simulink model "P702_NI_SoftECU"  (R2019a)
settings: Solver=ode1  StartTime=0.0  StopTime=Inf  FixedStep=0.001  RelTol=1e-3  EnableMultiTasking=on
PreLoadFcn:
  | run '.\VeriStand_BlockSet\NIVeriStandAddPaths.m'
undefined symbols (not defined in the file or in its folder): magnitude
libraries: simulink x83, simulink_extras x1
(part 41 of 76)

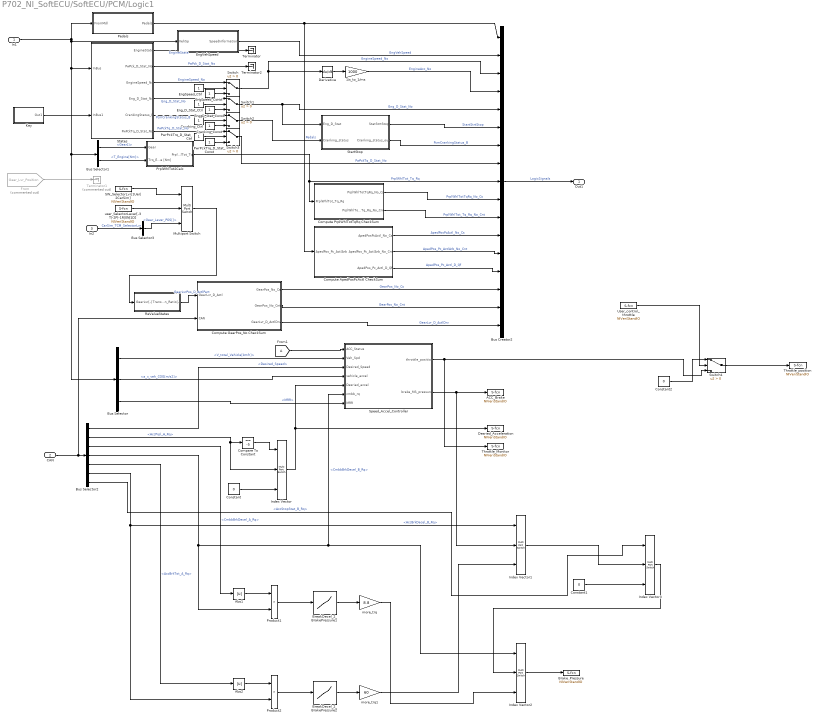
== system P702_NI_SoftECU/SoftECU/PCM/Logic1 ==
  In1 : Inport
  CAN : Inport  Port=2
  In2 : Inport  Port=3
  1/s_to_1/ms : Gain  Gain=1000
  ACC_Brake : S-Function  Priority=1  FunctionName=NIVeriStandIO  Parameters=width dtype portnum stime stype btype  SFunctionDeploymentMode=off  EnableBusSupport=off  mask(NI VeriStand Outport){portnum=1, width=-1, stime=-1, dtype=auto, stype=auto, btype=0}
      mask prompts: portnum "Port number:"; width "Port dimensions (-1 for dynamically sized):"; stime "Sample time (-1 for inherited):"; dtype "Data type:"; stype "Signal type:"; btype "Block type:"
      mask help: Use this outport on any level of nested subsystems to allow NI VeriStand software to map signals to it.
      mask init:
      | NIVeriStandIO_init;
      settings: CopyFcn=NIVeriStand_MDL_functions('', 'IO_copy');  DeleteFcn=NIVeriStand_MDL_functions('', 'IO_delete');  MoveFcn=set_param(gcb, 'Mask', 'on');
      mask Callback portnum: NIVeriStand_MDL_functions('', 'IO_setportnum');
      mask TypeOptions dtype: auto | double | single | int8 | uint8 | int16 | uint16 | int32 | uint32 | boolean
      mask Callback dtype: NIVeriStand_MDL_functions('', 'IO_booleansignal');
      mask TypeOptions stype: auto | real | complex
      mask Display:
      | patch([-x x], [-y y], [.90980 .81960 .32156]);
      | plot([xrad -x x xrad], [yrad -y y yrad]);
      | fprintf('NI Out%d', portnum);
  Abs1 : Abs
  Abs2 : Abs
  Brake_Pressure : S-Function  Priority=5  FunctionName=NIVeriStandIO  Parameters=width dtype portnum stime stype btype  SFunctionDeploymentMode=off  EnableBusSupport=off  mask(NI VeriStand Outport){portnum=5, width=-1, stime=-1, dtype=auto, stype=auto, btype=0}
      mask prompts: portnum "Port number:"; width "Port dimensions (-1 for dynamically sized):"; stime "Sample time (-1 for inherited):"; dtype "Data type:"; stype "Signal type:"; btype "Block type:"
      mask help: Use this outport on any level of nested subsystems to allow NI VeriStand software to map signals to it.
      mask init:
      | NIVeriStandIO_init;
      settings: CopyFcn=NIVeriStand_MDL_functions('', 'IO_copy');  DeleteFcn=NIVeriStand_MDL_functions('', 'IO_delete');  MoveFcn=set_param(gcb, 'Mask', 'on');
      mask Callback portnum: NIVeriStand_MDL_functions('', 'IO_setportnum');
      mask TypeOptions dtype: auto | double | single | int8 | uint8 | int16 | uint16 | int32 | uint32 | boolean
      mask Callback dtype: NIVeriStand_MDL_functions('', 'IO_booleansignal');
      mask TypeOptions stype: auto | real | complex
      mask Display:
      | patch([-x x], [-y y], [.90980 .81960 .32156]);
      | plot([xrad -x x xrad], [yrad -y y yrad]);
      | fprintf('NI Out%d', portnum);
  BreakDecel_2_BrakePressure1 : Lookup_n-D  NumberOfTableDimensions=1  BreakpointsForDimension1="[0   0.2  1   3.8   4.5    6     6.5   7   7.5   8   9   10    20]"  Table="[0   0.5    1   2       3     4      5      6   7     8    9   10   30]"  InternalRulePriority=Speed  RndMeth=Simplest  InputSameDT=on
  BreakDecel_2_BrakePressure2 : Lookup_n-D  NumberOfTableDimensions=1  BreakpointsForDimension1="[0   0.2  3.7   3.8   4.5    6     6.5   7   7.5   8   9   10    20]"  Table="[0   0    1   2       3     4      5      6   7     8    9   10   30]"  InternalRulePriority=Speed  RndMeth=Simplest  InputSameDT=on
  Bus Creator2 : BusCreator  Inputs=17
  Bus Selector : BusSelector  OutputSignals=V_total_Vehicle[km/h],a_x_veh_COG[m/s2],MRR
  Bus Selector1 : BusSelector  OutputSignals=Gear[],T_Engine[Nm]
  Bus Selector2 : BusSelector  OutputSignals=RealPCM.user_channel.Desired_Speed,ADAS.ACCDATA.AccPrpl_A_Rq,ADAS.ACCDATA_2.CmbbBrkDecel_A_Rq,ADAS.ACCDATA_2.CmbbBrkDecel_B_Rq,ADAS.ACCDATA.AccBrkTot_A_Rq,ADAS.ACCDATA.AccBrkDecel_B_Rq,ADAS.ACCDATA.AccStopStat_B_Rq
  Bus Selector3 : BusSelector  OutputSignals=Gear_Lever_POS[]
  Compare To Constant : simulink/Logic and Bit Operations/Compare To Constant  relop===  const=-5  OutDataTypeStr=boolean
  Compute ApedPosPcActl CheckSum : Subsystem
  Compute GearPos_No CheckSum : Subsystem
  Compute PrplWhlTotTqRq CheckSum : Subsystem
  Constant : Constant  Value=0
  Constant1 : Constant  Value=0
  Constant2 : Constant  Value=0
  Cranking_Const : Constant
  Cranking_Ctrl : Constant
  Derivative : Derivative
  Desried_Acceleration : S-Function  Priority=3  FunctionName=NIVeriStandIO  Parameters=width dtype portnum stime stype btype  SFunctionDeploymentMode=off  EnableBusSupport=off  mask(NI VeriStand Outport){portnum=3, width=-1, stime=-1, dtype=auto, stype=auto, btype=0}
      mask prompts: portnum "Port number:"; width "Port dimensions (-1 for dynamically sized):"; stime "Sample time (-1 for inherited):"; dtype "Data type:"; stype "Signal type:"; btype "Block type:"
      mask help: Use this outport on any level of nested subsystems to allow NI VeriStand software to map signals to it.
      mask init:
      | NIVeriStandIO_init;
      settings: CopyFcn=NIVeriStand_MDL_functions('', 'IO_copy');  DeleteFcn=NIVeriStand_MDL_functions('', 'IO_delete');  MoveFcn=set_param(gcb, 'Mask', 'on');
      mask Callback portnum: NIVeriStand_MDL_functions('', 'IO_setportnum');
      mask TypeOptions dtype: auto | double | single | int8 | uint8 | int16 | uint16 | int32 | uint32 | boolean
      mask Callback dtype: NIVeriStand_MDL_functions('', 'IO_booleansignal');
      mask TypeOptions stype: auto | real | complex
      mask Display:
      | patch([-x x], [-y y], [.90980 .81960 .32156]);
      | plot([xrad -x x xrad], [yrad -y y yrad]);
      | fprintf('NI Out%d', portnum);
  EngSpeed_Const : Constant
  EngSpeed_Ctrl : Constant
  EngVehSpeed : Subsystem
  Eng_D_Stat_Const : Constant
  Eng_D_Stat_Ctrl : Constant
  From : From  Commented=on  GotoTag=Gear_Lvr_Position  TagVisibility=global
  Index Vector{,1..3} (4 alike) : MultiPortSwitch  DataPortOrder=Zero-based contiguous  Inputs=2  zeroidx=on
  Key : Subsystem
      mask Display: disp('Key')
  Multiport Switch : MultiPortSwitch  Inputs=2
  Pedals : Subsystem
  Product1 : Product
  Product2 : Product
  PrplWhlTot2Calc : Subsystem
  PwrPckTrq_D_Stat_Const : Constant
  PwrPckTrq_D_Stat_Ctrl : Constant
  ReValueStates : Subsystem
      mask Display: disp('RevalueStates')
  SW_SelectorLvr[1Uer|2CarSim] : S-Function  Priority=2  FunctionName=NIVeriStandIO  Parameters=width dtype portnum stime stype btype  SFunctionDeploymentMode=off  EnableBusSupport=off  mask(NI VeriStand Inport){portnum=2, width=-1, stime=-1, dtype=auto, stype=auto, btype=1}
      mask prompts: portnum "Port number:"; width "Port dimensions (-1 for dynamically sized):"; stime "Sample time (-1 for inherited):"; dtype "Data type:"; stype "Signal type:"; btype "Block type:"
      mask help: Use this inport on any level of nested subsystems to allow NI VeriStand software to map signals to it.
      mask init:
      | NIVeriStandIO_init;
      settings: CopyFcn=NIVeriStand_MDL_functions('', 'IO_copy');  DeleteFcn=NIVeriStand_MDL_functions('', 'IO_delete');  MoveFcn=set_param(gcb, 'Mask', 'on');
      mask Callback portnum: NIVeriStand_MDL_functions('', 'IO_setportnum');
      mask TypeOptions dtype: auto | double | single | int8 | uint8 | int16 | uint16 | int32 | uint32 | boolean
      mask Callback dtype: NIVeriStand_MDL_functions('', 'IO_booleansignal');
      mask TypeOptions stype: auto | real | complex
      mask Display:
      | patch([-x x], [-y y], [.90980 .81960 .32156]);
      | plot([xrad -x x xrad], [yrad -y y yrad]);
      | fprintf('NI In%d', portnum);
  Speed_Accel_Controller : Subsystem
  StartStop : Subsystem
  States : Subsystem
  Switch{,1..4} (5 alike) : Switch  Criteria=u2 > Threshold
  Terminator : Terminator
  Terminator1 : Terminator  Commented=on
  Terminator2 : Terminator
  Throttle_Monitor : S-Function  Priority=4  FunctionName=NIVeriStandIO  Parameters=width dtype portnum stime stype btype  SFunctionDeploymentMode=off  EnableBusSupport=off  mask(NI VeriStand Outport){portnum=4, width=-1, stime=-1, dtype=auto, stype=auto, btype=0}
      mask prompts: portnum "Port number:"; width "Port dimensions (-1 for dynamically sized):"; stime "Sample time (-1 for inherited):"; dtype "Data type:"; stype "Signal type:"; btype "Block type:"
      mask help: Use this outport on any level of nested subsystems to allow NI VeriStand software to map signals to it.
      mask init:
      | NIVeriStandIO_init;
      settings: CopyFcn=NIVeriStand_MDL_functions('', 'IO_copy');  DeleteFcn=NIVeriStand_MDL_functions('', 'IO_delete');  MoveFcn=set_param(gcb, 'Mask', 'on');
      mask Callback portnum: NIVeriStand_MDL_functions('', 'IO_setportnum');
      mask TypeOptions dtype: auto | double | single | int8 | uint8 | int16 | uint16 | int32 | uint32 | boolean
      mask Callback dtype: NIVeriStand_MDL_functions('', 'IO_booleansignal');
      mask TypeOptions stype: auto | real | complex
      mask Display:
      | patch([-x x], [-y y], [.90980 .81960 .32156]);
      | plot([xrad -x x xrad], [yrad -y y yrad]);
      | fprintf('NI Out%d', portnum);
  Throttle_position : S-Function  Priority=2  FunctionName=NIVeriStandIO  Parameters=width dtype portnum stime stype btype  SFunctionDeploymentMode=off  EnableBusSupport=off  mask(NI VeriStand Outport){portnum=2, width=-1, stime=-1, dtype=auto, stype=auto, btype=0}
      mask prompts: portnum "Port number:"; width "Port dimensions (-1 for dynamically sized):"; stime "Sample time (-1 for inherited):"; dtype "Data type:"; stype "Signal type:"; btype "Block type:"
      mask help: Use this outport on any level of nested subsystems to allow NI VeriStand software to map signals to it.
      mask init:
      | NIVeriStandIO_init;
      settings: CopyFcn=NIVeriStand_MDL_functions('', 'IO_copy');  DeleteFcn=NIVeriStand_MDL_functions('', 'IO_delete');  MoveFcn=set_param(gcb, 'Mask', 'on');
      mask Callback portnum: NIVeriStand_MDL_functions('', 'IO_setportnum');
      mask TypeOptions dtype: auto | double | single | int8 | uint8 | int16 | uint16 | int32 | uint32 | boolean
      mask Callback dtype: NIVeriStand_MDL_functions('', 'IO_booleansignal');
      mask TypeOptions stype: auto | real | complex
      mask Display:
      | patch([-x x], [-y y], [.90980 .81960 .32156]);
      | plot([xrad -x x xrad], [yrad -y y yrad]);
      | fprintf('NI Out%d', portnum);
  User_control_throttle : S-Function  Priority=3  FunctionName=NIVeriStandIO  Parameters=width dtype portnum stime stype btype  SFunctionDeploymentMode=off  EnableBusSupport=off  mask(NI VeriStand Inport){portnum=3, width=-1, stime=-1, dtype=auto, stype=auto, btype=1}
      mask prompts: portnum "Port number:"; width "Port dimensions (-1 for dynamically sized):"; stime "Sample time (-1 for inherited):"; dtype "Data type:"; stype "Signal type:"; btype "Block type:"
      mask help: Use this inport on any level of nested subsystems to allow NI VeriStand software to map signals to it.
      mask init:
      | NIVeriStandIO_init;
      settings: CopyFcn=NIVeriStand_MDL_functions('', 'IO_copy');  DeleteFcn=NIVeriStand_MDL_functions('', 'IO_delete');  MoveFcn=set_param(gcb, 'Mask', 'on');
      mask Callback portnum: NIVeriStand_MDL_functions('', 'IO_setportnum');
      mask TypeOptions dtype: auto | double | single | int8 | uint8 | int16 | uint16 | int32 | uint32 | boolean
      mask Callback dtype: NIVeriStand_MDL_functions('', 'IO_booleansignal');
      mask TypeOptions stype: auto | real | complex
      mask Display:
      | patch([-x x], [-y y], [.90980 .81960 .32156]);
      | plot([xrad -x x xrad], [yrad -y y yrad]);
      | fprintf('NI In%d', portnum);
  more_trq : Gain  Gain=8.8
  more_trq1 : Gain  Gain=60
  user_SelectorLever[-3T|-2P|-1R|0N|1D] : S-Function  Priority=1  FunctionName=NIVeriStandIO  Parameters=width dtype portnum stime stype btype  SFunctionDeploymentMode=off  EnableBusSupport=off  mask(NI VeriStand Inport){portnum=1, width=-1, stime=-1, dtype=auto, stype=auto, btype=1}
      mask prompts: portnum "Port number:"; width "Port dimensions (-1 for dynamically sized):"; stime "Sample time (-1 for inherited):"; dtype "Data type:"; stype "Signal type:"; btype "Block type:"
      mask help: Use this inport on any level of nested subsystems to allow NI VeriStand software to map signals to it.
      mask init:
      | NIVeriStandIO_init;
      settings: CopyFcn=NIVeriStand_MDL_functions('', 'IO_copy');  DeleteFcn=NIVeriStand_MDL_functions('', 'IO_delete');  MoveFcn=set_param(gcb, 'Mask', 'on');
      mask Callback portnum: NIVeriStand_MDL_functions('', 'IO_setportnum');
      mask TypeOptions dtype: auto | double | single | int8 | uint8 | int16 | uint16 | int32 | uint32 | boolean
      mask Callback dtype: NIVeriStand_MDL_functions('', 'IO_booleansignal');
      mask TypeOptions stype: auto | real | complex
      mask Display:
      | patch([-x x], [-y y], [.90980 .81960 .32156]);
      | plot([xrad -x x xrad], [yrad -y y yrad]);
      | fprintf('NI In%d', portnum);
  Out1 : Outport
  wires:
  Key/1(Out1) -> States/2(InBus1)
  ReValueStates/1(Transmission_Ratio[-]) -> Compute GearPos_No CheckSum/1(GearLvr_D_Actl)  "GearLvrPos_D_ActlPart"
  From/1 -> Terminator1/1
  Switch3/1 -> Bus Creator2/8  "PwPckTq_D_Stat_No"
  States/6(PwPckTq_D_Stat_No) -> Switch3/1  "PwPckTq_D_Stat_No"
  PwrPckTrq_D_Stat_Ctrl/1 -> Switch3/2
  PwrPckTrq_D_Stat_Const/1 -> Switch3/3
  Switch2/1 -> StartStop/2(Cranking_status)
  Cranking_Ctrl/1 -> Switch2/2
  Cranking_Const/1 -> Switch2/3
  Eng_D_Stat_Ctrl/1 -> Switch1/2
  Eng_D_Stat_Const/1 -> Switch1/3
  Switch1/1 -> StartStop/1(Eng_D_Stat), Bus Creator2/5  "Eng_D_Stat_No"
  EngSpeed_Ctrl/1 -> Switch/2
  EngSpeed_Const/1 -> Switch/3
  Switch/1 -> Bus Creator2/3, Derivative/1  "EngineSpeed_No"
  States/5(CrankingStatus_B) -> Switch2/1  "PcmCrankingStatus_B"
  States/4(Eng_D_Stat_No) -> Switch1/1  "Eng_D_Stat_No"
  States/3(EngineSpeed_No) -> Switch/1  "EngineSpeed_No"
  PrplWhlTot2Calc/1(PrplWhlTot_Tq) -> Compute PrplWhlTotTqRq CheckSum/1(PrplWhlTot_Tq_Rq), Bus Creator2/9  "PrplWhlTot_Tq_Rq"
  Bus Selector1/2 -> PrplWhlTot2Calc/2(Trq_Engine [Nm])  "<T_Engine[Nm]>"
  Bus Selector1/1 -> PrplWhlTot2Calc/1(Gear)  "<Gear[]>"
  In1/1 -> Bus Selector/1, Bus Selector1/1, States/1(InBus), EngVehSpeed/1(VehSp), Pedals/1(FromMdl)
  EngVehSpeed/1(SpeedInformation) -> Bus Creator2/2  "EngVehSpeed"
  Pedals/1(Pedals) -> Compute ApedPosPcActl CheckSum/1(ApedPos_Pc_ActlArb), Bus Creator2/1  "Pedals"
  StartStop/2(Cranking_status_out) -> Bus Creator2/7  "PcmCrankingStatus_B"
  StartStop/1(StatStrtStop) -> Bus Creator2/6  "StartStrtStop"
  1/s_to_1/ms/1 -> Bus Creator2/4  "EngineAcc_No"
  Derivative/1 -> 1/s_to_1/ms/1
  Bus Creator2/1 -> Out1/1  "LogicSignals"
  States/2("PwPck_D_Stat_No ") -> Terminator2/1  "PwPck_D_Stat_No"
  States/1(EngineState) -> Terminator/1  "EngineState"
  Compute PrplWhlTotTqRq CheckSum/1(PrplWhlTotTqRq_No_Cs) -> Bus Creator2/10  "PrplWhlTotTqRq_No_Cs"
  Compute ApedPosPcActl CheckSum/1(ApedPosPcActl_No_Cs) -> Bus Creator2/12  "ApedPosPcActl_No_Cs"
  Compute PrplWhlTotTqRq CheckSum/2(PrplWhlTot_Tq_Rq_No_Cnt) -> Bus Creator2/11  "PrplWhlTot_Tq_Rq_No_Cnt"
  Compute ApedPosPcActl CheckSum/3(ApedPos_Pc_Actl_D_Qf) -> Bus Creator2/14  "ApedPos_Pc_Actl_D_Qf"
  Compute ApedPosPcActl CheckSum/2(ApedPos_Pc_ActlArb_No_Cnt) -> Bus Creator2/13  "ApedPos_Pc_ActlArb_No_Cnt"
  Compute GearPos_No CheckSum/3(GearLvr_D_ActlDrv) -> Bus Creator2/17  "GearLvr_D_ActlDrv"
  Compute GearPos_No CheckSum/2(GearPos_No_Cnt) -> Bus Creator2/16  "GearPos_No_Cnt"
  Compute GearPos_No CheckSum/1(GearPos_No_Cs) -> Bus Creator2/15  "GearPos_No_Cs"
  CAN/1 -> Compute GearPos_No CheckSum/2(CAN), Bus Selector2/1
  Speed_Accel_Controller/1(throttle_position) -> Switch4/3, Throttle_Monitor/1
  Bus Selector/1 -> Speed_Accel_Controller/2(Veh_Spd)  "<V_total_Vehicle[km/h]>"
  Bus Selector2/1 -> Speed_Accel_Controller/3(Desired_Speed)  "<Desired_Speed>"
  Bus Selector/2 -> Speed_Accel_Controller/4(vehicle_accel)  "<a_x_veh_COG[m/s2]>"
  [A] -> Speed_Accel_Controller/1(ACC_Status)
  Bus Selector2/5 -> Abs2/1  "<AccBrkTot_A_Rq>"
  Bus Selector2/2 -> Index Vector/2, Compare To Constant/1  "<AccPrpl_A_Rq>"
  Compare To Constant/1 -> Index Vector/1
  Constant/1 -> Index Vector/3
  Index Vector/1 -> Speed_Accel_Controller/5(Desried_accel), Desried_Acceleration/1
  Speed_Accel_Controller/2(brake_MS_pressure) -> Index Vector1/2, ACC_Brake/1
  Bus Selector2/4 -> Speed_Accel_Controller/6(cmbb_rq), Index Vector2/1, Product1/2  "<CmbbBrkDecel_B_Rq>"
  BreakDecel_2_BrakePressure1/1 -> more_trq/1
  Product1/1 -> BreakDecel_2_BrakePressure1/1
  Abs1/1 -> Product1/1
  Bus Selector2/3 -> Abs1/1  "<CmbbBrkDecel_A_Rq>"
  BreakDecel_2_BrakePressure2/1 -> more_trq1/1
  Product2/1 -> BreakDecel_2_BrakePressure2/1
  Abs2/1 -> Product2/1
  more_trq1/1 -> Index Vector1/3
  Bus Selector2/6 -> Index Vector1/1, Product2/2  "<AccBrkDecel_B_Rq>"
  Index Vector3/1 -> Index Vector2/2
  more_trq/1 -> Index Vector2/3
  Index Vector2/1 -> Brake_Pressure/1
  Index Vector1/1 -> Index Vector3/2
  Bus Selector2/7 -> Index Vector3/1  "<AccStopStat_B_Rq>"
  Constant1/1 -> Index Vector3/3
  Constant2/1 -> Switch4/1
  Switch4/1 -> Throttle_position/1
  Bus Selector/3 -> Speed_Accel_Controller/7(MRR)  "<MRR>"
  user_SelectorLever[-3T|-2P|-1R|0N|1D]/1 -> Multiport Switch/2
  Multiport Switch/1 -> ReValueStates/1(GearLvr[-])
  SW_SelectorLvr[1Uer|2CarSim]/1 -> Multiport Switch/1
  In2/1 -> Bus Selector3/1  "CarSim_TCM_SelectorLvr"
  Bus Selector3/1 -> Multiport Switch/3  "<Gear_Lever_POS[]>"
  User_control_throttle/1 -> Switch4/2

== system P702_NI_SoftECU/SoftECU/PCM/Mapping ==
  In1 : Inport
  Bus Creator : BusCreator  Inputs=9
  EngBrakeData : Subsystem
  EngVehicleSpThrottle : Subsystem
  EngVehicleSpThrottle2 : Subsystem
  EngineClimateData : Subsystem
  EngineClutchData : Subsystem
  EngineData_7 : Subsystem
  PowertrainData_10 : Subsystem
  TorqueDataEngFlags : Subsystem
  VehicleOperatingModes : Subsystem
  Out1 : Outport
  wires:
  TorqueDataEngFlags/1(Out1) -> Bus Creator/8  "TorqueDataEngFlags"
  EngineData_7/1(Out1) -> Bus Creator/7  "EngineData_7"
  VehicleOperatingModes/1(Out1) -> Bus Creator/6  "VehicleOperatingModes"
  EngVehicleSpThrottle2/1(Out1) -> Bus Creator/5  "EngVehicleSpThottle2"
  EngVehicleSpThrottle/1(Out1) -> Bus Creator/4  "EngVehicleSpThrottle"
  EngineClutchData/1(Out1) -> Bus Creator/3  "EngineClutchData"
  EngineClimateData/1(Out1) -> Bus Creator/2  "EngineClimateData"
  EngBrakeData/1(Out1) -> Bus Creator/1  "EngBrakeData"
  Bus Creator/1 -> Out1/1  "MsgSignals"
  In1/1 -> EngBrakeData/1(In1), EngineClimateData/1(In1), EngineClutchData/1(In1), EngVehicleSpThrottle/1(In1), EngineData_7/1(In1), PowertrainData_10/1(In1), TorqueDataEngFlags/1(In1), VehicleOperatingModes/1(In1), EngVehicleSpThrottle2/1(In1)
  PowertrainData_10/1(Out1) -> Bus Creator/9  "PowertrainData_10"

== system P702_NI_SoftECU/SoftECU/PSCM/Logic ==
  In1 : Inport
  Bus Creator : BusCreator  Inputs=3
  Checksums : Subsystem
  Counters : Subsystem
  UnitConversion : Subsystem
  Out1 : Outport
  wires:
  In1/1 -> UnitConversion/1(In1)
  Bus Creator/1 -> Out1/1  "LogicSignals"
  UnitConversion/1(Out1) -> Bus Creator/1, Checksums/4(StePinRelCalib_Sns), Checksums/3(StePinComp_Est), Checksums/2(StePinRelInit_Sns)
  Counters/1(Out1) -> Checksums/1(StePinAng_Counter), Bus Creator/2
  Checksums/1(Out1) -> Bus Creator/3

== system P702_NI_SoftECU/SoftECU/PSCM/Mapping ==
  In1 : Inport
  SteeringPinion_Data : Subsystem
  Out1 : Outport
  wires:
  SteeringPinion_Data/1(Out1) -> Out1/1
  In1/1 -> SteeringPinion_Data/1(In1)

== system P702_NI_SoftECU/SoftECU/RCM/Logic ==
  In1 : Inport
  Bus Creator : BusCreator  Inputs=4
  Bus Selector : BusSelector  OutputSignals=RollRate_Vehicle_CoG[rad|s],YawRate_Vehicle_CoG[rad|s],a_y_Vehicle_CoG[m|s2],a_x_Vehicle_CoG[m|s2],a_z_Vehicle_CoG[m|s2]
  Bus Selector1 : BusSelector  OutputSignals=RollYawCounter,AccelCounter
  Checksums : Subsystem
  Counters : Subsystem
  StatusMessage : Subsystem
  UnitConversion : Subsystem
  Out1 : Outport
  wires:
  In1/1 -> UnitConversion/1(In1), StatusMessage/1(In1)
  Bus Creator/1 -> Out1/1  "LogicSignals"
  UnitConversion/1(Out1) -> Bus Selector/1, Bus Creator/1
  StatusMessage/1(Out1) -> Bus Creator/2
  Counters/1(Out1) -> Bus Creator/3, Bus Selector1/1
  Checksums/1(Out1) -> Bus Creator/4
  Bus Selector/1 -> Checksums/3(RollRate)  "<RollRate_Vehicle_CoG[rad|s]>"
  Bus Selector/2 -> Checksums/4(YawRate)  "<YawRate_Vehicle_CoG[rad|s]>"
  Bus Selector1/1 -> Checksums/1(Counter)  "<RollYawCounter>"
  Bus Selector1/2 -> Checksums/2(Accel_Counter)  "<AccelCounter>"
  Bus Selector/4 -> Checksums/6(LongAccel)  "<a_x_Vehicle_CoG[m|s2]>"
  Bus Selector/3 -> Checksums/5(LatAccel)  "<a_y_Vehicle_CoG[m|s2]>"
  Bus Selector/5 -> Checksums/7(VertAccel)  "<a_z_Vehicle_CoG[m|s2]>"

== system P702_NI_SoftECU/SoftECU/RCM/Mapping ==
  In1 : Inport
  Accel_Data : Subsystem
  Bus Creator : BusCreator  Inputs=3
  RCMStatusMessage2 : Subsystem
  Yaw_Data : Subsystem
  Out1 : Outport
  wires:
  Bus Creator/1 -> Out1/1  "MsgSignals"
  In1/1 -> Accel_Data/1(In1), Yaw_Data/1(In1), RCMStatusMessage2/1(In1)
  Accel_Data/1(Out1) -> Bus Creator/1  "Accel_Data"
  Yaw_Data/1(Out1) -> Bus Creator/2  "Yaw_Data"
  RCMStatusMessage2/1(Out1) -> Bus Creator/3

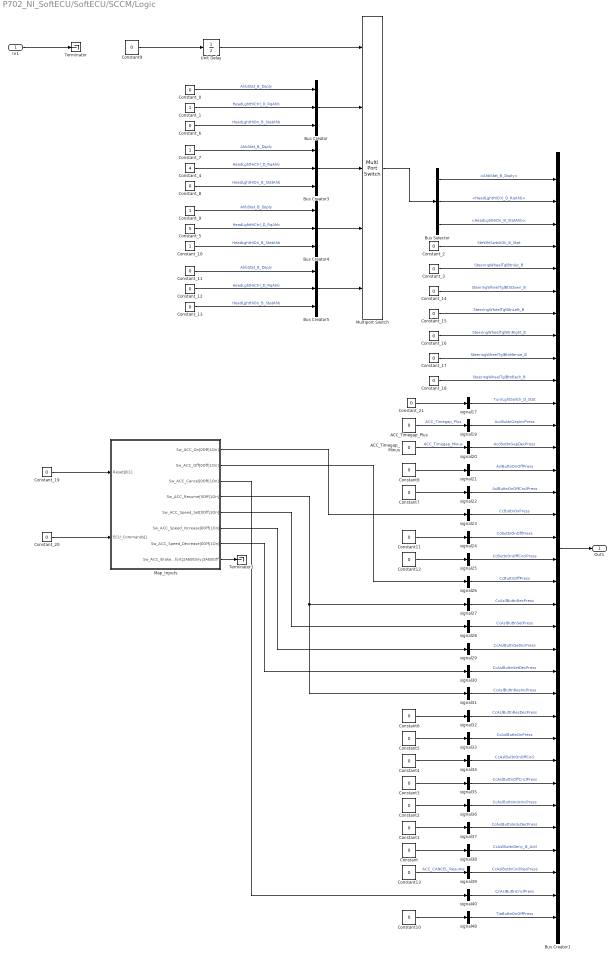
== system P702_NI_SoftECU/SoftECU/SCCM/Logic ==
  In1 : Inport
  ACC_Timegap_Minus : Constant  Value=0
  ACC_Timegap_Plus : Constant  Value=0
  Bus Creator{,3..5} (4 alike) : BusCreator  Inputs=3
  Bus Creator1 : BusCreator  Inputs=34
  Bus Selector : BusSelector  OutputSignals=AhbStat_B_Dsply,HeadLghtHiCtrl_D_RqAhb,HeadLghtHiOn_B_StatAhb
  Constant{,1..9,11..13} (13 alike) : Constant  Value=0
  Constant10 : Constant  Value=0  OutDataTypeStr=boolean
  Constant_{0,2..3,6,8,11..21} (16 alike) : Constant  Value=0
  Constant_{1,7,9..10} (4 alike) : Constant
  Constant_4 : Constant  Value=4
  Constant_5 : Constant  Value=5
  Map_Inputs : Subsystem
  Multiport Switch : MultiPortSwitch  DataPortOrder=Zero-based contiguous  Inputs=4  zeroidx=on
  Terminator : Terminator
  Terminator1 : Terminator
  Unit Delay : UnitDelay  SampleTime=-1  HasFrameUpgradeWarning=on
  signal{17,19..40,48} (24 alike) : Demux  Outputs=1
  Out1 : Outport
  wires:
  Constant9/1 -> Unit Delay/1
  Constant_0/1 -> Bus Creator/1  "AhbStat_B_Dsply"
  Constant_1/1 -> Bus Creator/2  "HeadLghtHiCtrl_D_RqAhb"
  Constant_6/1 -> Bus Creator/3  "HeadLghtHiOn_B_StatAhb"
  Bus Creator/1 -> Multiport Switch/2
  Constant_7/1 -> Bus Creator3/1  "AhbStat_B_Dsply"
  Constant_4/1 -> Bus Creator3/2  "HeadLghtHiCtrl_D_RqAhb"
  Constant_8/1 -> Bus Creator3/3  "HeadLghtHiOn_B_StatAhb"
  Bus Creator3/1 -> Multiport Switch/3
  Constant_9/1 -> Bus Creator4/1  "AhbStat_B_Dsply"
  Constant_5/1 -> Bus Creator4/2  "HeadLghtHiCtrl_D_RqAhb"
  Constant_10/1 -> Bus Creator4/3  "HeadLghtHiOn_B_StatAhb"
  Bus Creator4/1 -> Multiport Switch/4
  Constant_11/1 -> Bus Creator5/1  "AhbStat_B_Dsply"
  Constant_12/1 -> Bus Creator5/2  "HeadLghtHiCtrl_D_RqAhb"
  Constant_13/1 -> Bus Creator5/3  "HeadLghtHiOn_B_StatAhb"
  Bus Creator5/1 -> Multiport Switch/5
  Unit Delay/1 -> Multiport Switch/1
  Multiport Switch/1 -> Bus Selector/1
  Bus Selector/1 -> Bus Creator1/1  "<AhbStat_B_Dsply>"
  Bus Selector/2 -> Bus Creator1/2  "<HeadLghtHiCtrl_D_RqAhb>"
  Bus Selector/3 -> Bus Creator1/3  "<HeadLghtHiOn_B_StatAhb>"
  Bus Creator1/1 -> Out1/1
  Constant_2/1 -> Bus Creator1/4  "SteWhlSwtchOk_B_Stat"
  Constant_3/1 -> Bus Creator1/5  "SteeringWheelTglBtnUp_B"
  Constant_15/1 -> Bus Creator1/7  "SteeringWheelTglBtnLeft_B"
  Constant_16/1 -> Bus Creator1/8  "SteeringWheelTglBtnRight_B"
  Constant_17/1 -> Bus Creator1/9  "SteeringWheelTglBtnMenue_B"
  Constant_18/1 -> Bus Creator1/10  "SteeringWheelTglBtnBack_B"
  Constant_14/1 -> Bus Creator1/6  "SteeringWheelTglBtnDown_B"
  Constant10/1 -> signal48/1
  signal48/1 -> Bus Creator1/34  "TjaButtnOnOffPress"
  In1/1 -> Terminator/1
  signal40/1 -> Bus Creator1/33  "CcAslButtnCnclPress"
  signal39/1 -> Bus Creator1/32  "CcAslButtnCnclResPress"
  Constant/1 -> signal38/1
  signal38/1 -> Bus Creator1/31  "CcAslButtnDeny_B_Actl"
  Constant1/1 -> signal37/1
  signal37/1 -> Bus Creator1/30  "CcAslButtnIndxDecPress"
  Constant2/1 -> signal36/1
  signal36/1 -> Bus Creator1/29  "CcAslButtnIndxIncPress"
  Constant3/1 -> signal35/1
  signal35/1 -> Bus Creator1/28  "CcAslButtnOffCnclPress"
  Constant4/1 -> signal34/1
  signal34/1 -> Bus Creator1/27  "CcAslButtnOnOffCncl"
  Constant5/1 -> signal33/1
  signal33/1 -> Bus Creator1/26  "CcAslButtnOnPress"
  Constant6/1 -> signal32/1
  signal32/1 -> Bus Creator1/25  "CcAslButtnResDecPress"
  signal31/1 -> Bus Creator1/24  "CcAslButtnResIncPress"
  signal30/1 -> Bus Creator1/23  "CcAslButtnSetDecPress"
  signal29/1 -> Bus Creator1/22  "CcAslButtnSetIncPress"
  Map_Inputs/5(Sw_ACC_Speed_Set[0Off|1On]) -> signal28/1
  signal28/1 -> Bus Creator1/21  "CcAslButtnSetPress"
  signal27/1 -> Bus Creator1/20  "CcAsllButtnResPress"
  signal26/1 -> Bus Creator1/19  "CcButtnOffPress"
  signal25/1 -> Bus Creator1/18  "CcButtnOnOffCnclPress"
  Constant7/1 -> signal22/1
  Constant8/1 -> signal21/1
  Constant_21/1 -> signal17/1
  ACC_Timegap_Plus/1 -> signal19/1  "ACC_Timegap_Plus"
  Map_Inputs/1(Sw_ACC_On[0Off|1On]) -> signal23/1
  Constant11/1 -> signal24/1
  Map_Inputs/2(Sw_ACC_Off[0Off|1On]) -> signal26/1
  Map_Inputs/4(Sw_ACC_Resume[0Off|1On]) -> signal27/1, signal31/1
  Map_Inputs/6(Sw_ACC_Speed_Increase[0Off|1On]) -> signal29/1
  Map_Inputs/7(Sw_ACC_Speed_Decrease[0Off|1On]) -> signal30/1
  Constant13/1 -> signal39/1  "ACC_CANCEL_Resume"
  Map_Inputs/3(Sw_ACC_Cancel[0Off|1On]) -> signal40/1
  signal24/1 -> Bus Creator1/17  "CcButtnOnOffPress"
  signal23/1 -> Bus Creator1/16  "CcButtnOnPress"
  signal22/1 -> Bus Creator1/15  "AslButtnOnOffCnclPress"
  signal21/1 -> Bus Creator1/14  "AslButtnOnOffPress"
  signal20/1 -> Bus Creator1/13  "AccButtnGapDecPress"
  signal19/1 -> Bus Creator1/12  "AccButtnGapIncPress"
  signal17/1 -> Bus Creator1/11  "TurnLghtSwtch_D_Stat"
  Constant_19/1 -> Map_Inputs/1(Reset[0|1])
  Constant_20/1 -> Map_Inputs/2(ECU_Commands[])
  Constant12/1 -> signal25/1
  Map_Inputs/8(Sw_ACC_BrakeMode[1Comfort|2AEBOnly|3AEBOff]) -> Terminator1/1
  ACC_Timegap_Minus/1 -> signal20/1  "ACC_Timegap_Minus"

== system P702_NI_SoftECU/SoftECU/SCCM/Mapping ==
  In1 : Inport
  Bus Creator1 : BusCreator  Inputs=2
  Steering_Data : Subsystem
  Steering_Wheel_Data2 : Subsystem
  Out1 : Outport
  wires:
  Bus Creator1/1 -> Out1/1  "MsgSignals"
  In1/1 -> Steering_Wheel_Data2/1(In1), Steering_Data/1(In1)
  Steering_Data/1(Out1) -> Bus Creator1/1  "Steering_Data"
  Steering_Wheel_Data2/1(Out1) -> Bus Creator1/2  "Steering_Wheel_Data2"

== system P702_NI_SoftECU/SoftECU/SRR_L/Carsim_L ==
  note: Position in Carsim Coordinate
      | X: forward
      | Y: left
      | Lhan18
  Bus Creator : BusCreator  Inputs=3
  Gain1 : Gain  Gain=pi/180
  x_offset : Constant  Value=-1.5
  y_offset : Constant  Value=0.8
  yaw_head : Constant  Value=90
  CSP : Outport
  wires:
  Bus Creator/1 -> CSP/1  "Position"
  x_offset/1 -> Bus Creator/1  "c_sensor_x"
  y_offset/1 -> Bus Creator/2  "c_sensor_y"
  yaw_head/1 -> Gain1/1
  Gain1/1 -> Bus Creator/3  "c_sensor_yaw"

== system P702_NI_SoftECU/SoftECU/SRR_L/FrontLeft_SOD ==
  In1 : Inport
  Sensor_pos : Inport  Port=2
  CSP : Inport  Port=3
  Bus Creator : BusCreator  Inputs=4
  Bus Creator1 : BusCreator  Inputs=4
  Bus Creator2 : BusCreator  Inputs=4
  Bus Creator3 : BusCreator  Inputs=3
  Bus Selector : BusSelector  OutputSignals=SRR_L_DET_RANGE_01[m],SRR_L_DET_AZIMUTH_01[rad],SRR_L_DET_RANGE_RATE_01[m/s],SRR_L_DET_ELEVATION_01[rad]
  Bus Selector1 : BusSelector  OutputSignals=SRR_L_DET_RANGE_02[m],SRR_L_DET_AZIMUTH_02[rad],SRR_L_DET_RANGE_RATE_02[m/s],SRR_L_DET_ELEVATION_02[rad]
  Bus Selector2 : BusSelector  OutputSignals=SRR_L_DET_RANGE_03[m],SRR_L_DET_AZIMUTH_03[rad],SRR_L_DET_RANGE_RATE_03[m/s],SRR_L_DET_ELEVATION_03[rad]
  SRR_FL_001 : Subsystem
  SRR_FL_002 : Subsystem
  SRR_FL_003 : Subsystem
  FL_SOD : Outport
  wires:
  CSP/1 -> SRR_FL_002/3(CSP), SRR_FL_003/3(CSP), SRR_FL_001/3(CSP)
  Sensor_pos/1 -> SRR_FL_001/2(sensor_pos), SRR_FL_002/2(sensor_pos), SRR_FL_003/2(sensor_pos)
  Bus Creator2/1 -> SRR_FL_003/1(target_pos)  "<Carsim_det_003>"
  Bus Selector2/4 -> Bus Creator2/4  "<SRR_L_DET_ELEVATION_03[rad]>"
  Bus Selector2/3 -> Bus Creator2/3  "<SRR_L_DET_RANGE_RATE_03[m/s]>"
  Bus Selector1/4 -> Bus Creator1/4  "<SRR_L_DET_ELEVATION_02[rad]>"
  SRR_FL_002/1(SRR_FL_002) -> Bus Creator3/2  "SRR_FL_002"
  SRR_FL_001/1(SRR_FL_001) -> Bus Creator3/1  "SRR_FL_001"
  In1/1 -> Bus Selector/1, Bus Selector1/1, Bus Selector2/1
  Bus Selector2/1 -> Bus Creator2/1  "<SRR_L_DET_RANGE_03[m]>"
  Bus Selector1/2 -> Bus Creator1/2  "<SRR_L_DET_AZIMUTH_02[rad]>"
  Bus Selector2/2 -> Bus Creator2/2  "<SRR_L_DET_AZIMUTH_03[rad]>"
  Bus Selector1/1 -> Bus Creator1/1  "<SRR_L_DET_RANGE_02[m]>"
  Bus Selector/3 -> Bus Creator/3  "<SRR_L_DET_RANGE_RATE_01[m/s]>"
  Bus Selector/4 -> Bus Creator/4  "<SRR_L_DET_ELEVATION_01[rad]>"
  Bus Selector/1 -> Bus Creator/1  "<SRR_L_DET_RANGE_01[m]>"
  Bus Selector/2 -> Bus Creator/2  "<SRR_L_DET_AZIMUTH_01[rad]>"
  Bus Creator/1 -> SRR_FL_001/1(target_pos)  "<Carsim_det_001>"
  Bus Selector1/3 -> Bus Creator1/3  "<SRR_L_DET_RANGE_RATE_02[m/s]>"
  Bus Creator1/1 -> SRR_FL_002/1(target_pos)  "<Carsim_det_002>"
  Bus Creator3/1 -> FL_SOD/1
  SRR_FL_003/1(SRR_FL_003) -> Bus Creator3/3  "SRR_FL_003"

== system P702_NI_SoftECU/SoftECU/SRR_L/RearLeft_SOD ==
  In1 : Inport
  Sensor_pos : Inport  Port=2
  CSP : Inport  Port=3
  Bus Creator : BusCreator  Inputs=4
  Bus Creator1 : BusCreator  Inputs=4
  Bus Creator2 : BusCreator  Inputs=4
  Bus Creator3 : BusCreator  Inputs=3
  Bus Selector : BusSelector  OutputSignals=SRR_L_DET_RANGE_01[m],SRR_L_DET_AZIMUTH_01[rad],SRR_L_DET_RANGE_RATE_01[m/s],SRR_L_DET_ELEVATION_01[rad]
  Bus Selector1 : BusSelector  OutputSignals=SRR_L_DET_RANGE_02[m],SRR_L_DET_AZIMUTH_02[rad],SRR_L_DET_RANGE_RATE_02[m/s],SRR_L_DET_ELEVATION_02[rad]
  Bus Selector2 : BusSelector  OutputSignals=SRR_L_DET_RANGE_03[m],SRR_L_DET_AZIMUTH_03[rad],SRR_L_DET_RANGE_RATE_03[m/s],SRR_L_DET_ELEVATION_03[rad]
  "SRR_RL_001 " : Subsystem
  SRR_RL_002 : Subsystem
  SRR_RL_003 : Subsystem
  RL_SOD : Outport
  wires:
  Bus Creator1/1 -> SRR_RL_002/1(target_pos)  "<Carsim_det_002>"
  Bus Selector1/3 -> Bus Creator1/3  "<SRR_L_DET_RANGE_RATE_02[m/s]>"
  Bus Creator/1 -> "SRR_RL_001 "/1(target_pos)  "<Carsim_det_001>"
  Bus Selector/3 -> Bus Creator/3  "<SRR_L_DET_RANGE_RATE_01[m/s]>"
  Bus Selector/1 -> Bus Creator/1  "<SRR_L_DET_RANGE_01[m]>"
  Bus Selector/4 -> Bus Creator/4  "<SRR_L_DET_ELEVATION_01[rad]>"
  Bus Selector/2 -> Bus Creator/2  "<SRR_L_DET_AZIMUTH_01[rad]>"
  Bus Selector1/1 -> Bus Creator1/1  "<SRR_L_DET_RANGE_02[m]>"
  Bus Selector2/2 -> Bus Creator2/2  "<SRR_L_DET_AZIMUTH_03[rad]>"
  Bus Selector1/2 -> Bus Creator1/2  "<SRR_L_DET_AZIMUTH_02[rad]>"
  Bus Selector2/1 -> Bus Creator2/1  "<SRR_L_DET_RANGE_03[m]>"
  In1/1 -> Bus Selector2/1, Bus Selector1/1, Bus Selector/1
  SRR_RL_002/1(SRR_RL_002) -> Bus Creator3/2  "SRR_RL_002"
  Bus Selector1/4 -> Bus Creator1/4  "<SRR_L_DET_ELEVATION_02[rad]>"
  Bus Selector2/3 -> Bus Creator2/3  "<SRR_L_DET_RANGE_RATE_03[m/s]>"
  Bus Selector2/4 -> Bus Creator2/4  "<SRR_L_DET_ELEVATION_03[rad]>"
  Bus Creator2/1 -> SRR_RL_003/1(target_pos)  "<Carsim_det_003>"
  Sensor_pos/1 -> SRR_RL_003/2(sensor_pos), SRR_RL_002/2(sensor_pos), "SRR_RL_001 "/2(sensor_pos)
  CSP/1 -> "SRR_RL_001 "/3(CSP), SRR_RL_003/3(CSP), SRR_RL_002/3(CSP)
  Bus Creator3/1 -> RL_SOD/1
  "SRR_RL_001 "/1(SRR_RL_001) -> Bus Creator3/1  "SRR_RL_001"
  SRR_RL_003/1(SRR_RL_003) -> Bus Creator3/3  "SRR_RL_003"

== system P702_NI_SoftECU/SoftECU/SRR_L/SensorPosition_FL ==
  note: Position in Carsim Coordinate
      | X: forward
      | Y: left
      | Lhan18
  Bus Creator : BusCreator  Inputs=3
  Gain1 : Gain  Gain=pi/180
  x_offset : Constant  Value=0.5
  y_offset : Constant  Value=0.8
  yaw_head : Constant  Value=60
  SensorPosition : Outport
  wires:
  Bus Creator/1 -> SensorPosition/1  "Position"
  x_offset/1 -> Bus Creator/1  "sensor_x"
  y_offset/1 -> Bus Creator/2  "sensor_y"
  yaw_head/1 -> Gain1/1
  Gain1/1 -> Bus Creator/3  "sensor_yaw"

== system P702_NI_SoftECU/SoftECU/SRR_L/SensorPosition_RL ==
  note: Position in Carsim Coordinate
      | X: forward
      | Y: left
      | Lhan18
  Bus Creator : BusCreator  Inputs=3
  Gain : Gain  Gain=pi/180
  x_offset : Constant  Value=-3.5
  y_offset : Constant  Value=0.8
  yaw_head : Constant  Value=120
  SensorPosition : Outport
  wires:
  Bus Creator/1 -> SensorPosition/1  "Position"
  x_offset/1 -> Bus Creator/1  "sensor_x"
  y_offset/1 -> Bus Creator/2  "sensor_y"
  yaw_head/1 -> Gain/1
  Gain/1 -> Bus Creator/3  "sensor_yaw"

== system P702_NI_SoftECU/SoftECU/SRR_R/Carsim_R ==
  note: Position in Carsim Coordinate
      | X: forward
      | Y: left
      | Lhan18
  Bus Creator : BusCreator  Inputs=3
  Gain1 : Gain  Gain=pi/180
  x_offset : Constant  Value=-1.5
  y_offset : Constant  Value=-0.8
  yaw_head : Constant  Value=-90
  CSP : Outport
  wires:
  Bus Creator/1 -> CSP/1  "Position"
  x_offset/1 -> Bus Creator/1  "c_sensor_x"
  y_offset/1 -> Bus Creator/2  "c_sensor_y"
  yaw_head/1 -> Gain1/1
  Gain1/1 -> Bus Creator/3  "c_sensor_yaw"

== system P702_NI_SoftECU/SoftECU/SRR_R/FrontRight_SOD ==
  In1 : Inport
  Sensor_pos : Inport  Port=2
  CSP : Inport  Port=3
  Bus Creator : BusCreator  Inputs=4
  Bus Creator1 : BusCreator  Inputs=4
  Bus Creator2 : BusCreator  Inputs=4
  Bus Creator3 : BusCreator  Inputs=3
  Bus Selector : BusSelector  OutputSignals=SRR_R_DET_RANGE_01[m],SRR_R_DET_RANGE_RATE_01[m/s],SRR_R_DET_AZIMUTH_01[rad],SRR_R_DET_ELEVATION_01[rad]
  Bus Selector1 : BusSelector  OutputSignals=SRR_R_DET_RANGE_02[m],SRR_R_DET_RANGE_RATE_02[m/s],SRR_R_DET_AZIMUTH_02[rad],SRR_R_DET_ELEVATION_02[rad]
  Bus Selector2 : BusSelector  OutputSignals=SRR_R_DET_RANGE_03[m],SRR_R_DET_RANGE_RATE_03[m/s],SRR_R_DET_AZIMUTH_03[rad],SRR_R_DET_ELEVATION_03[rad]
  "SRR_FR_001 " : Subsystem
  SRR_FR_002 : Subsystem
  SRR_FR_003 : Subsystem
  FR_SOD : Outport
  wires:
  CSP/1 -> SRR_FR_002/3(CSP), SRR_FR_003/3(CSP), "SRR_FR_001 "/3(CSP)
  Sensor_pos/1 -> "SRR_FR_001 "/2(sensor_pos), SRR_FR_002/2(sensor_pos), SRR_FR_003/2(sensor_pos)
  Bus Creator2/1 -> SRR_FR_003/1(target_pos)  "<Carsim_det_003>"
  Bus Selector2/4 -> Bus Creator2/4  "<SRR_R_DET_ELEVATION_03[rad]>"
  Bus Selector2/3 -> Bus Creator2/3  "<SRR_R_DET_AZIMUTH_03[rad]>"
  Bus Selector1/4 -> Bus Creator1/4  "<SRR_R_DET_ELEVATION_02[rad]>"
  In1/1 -> Bus Selector/1, Bus Selector1/1, Bus Selector2/1
  Bus Selector2/1 -> Bus Creator2/1  "<SRR_R_DET_RANGE_03[m]>"
  Bus Selector1/2 -> Bus Creator1/2  "<SRR_R_DET_RANGE_RATE_02[m/s]>"
  Bus Selector2/2 -> Bus Creator2/2  "<SRR_R_DET_RANGE_RATE_03[m/s]>"
  Bus Selector1/1 -> Bus Creator1/1  "<SRR_R_DET_RANGE_02[m]>"
  Bus Selector/3 -> Bus Creator/3  "<SRR_R_DET_AZIMUTH_01[rad]>"
  Bus Selector/4 -> Bus Creator/4  "<SRR_R_DET_ELEVATION_01[rad]>"
  Bus Selector/1 -> Bus Creator/1  "<SRR_R_DET_RANGE_01[m]>"
  Bus Selector/2 -> Bus Creator/2  "<SRR_R_DET_RANGE_RATE_01[m/s]>"
  Bus Creator/1 -> "SRR_FR_001 "/1(target_pos)  "<Carsim_det_001>"
  Bus Selector1/3 -> Bus Creator1/3  "<SRR_R_DET_AZIMUTH_02[rad]>"
  Bus Creator1/1 -> SRR_FR_002/1(target_pos)  "<Carsim_det_002>"
  Bus Creator3/1 -> FR_SOD/1
  "SRR_FR_001 "/1(SRR_FR_001) -> Bus Creator3/1  "SRR_FR_001"
  SRR_FR_002/1(SRR_FR_002) -> Bus Creator3/2  "SRR_FR_002"
  SRR_FR_003/1(SRR_FR_003) -> Bus Creator3/3  "SRR_FR_003"

== system P702_NI_SoftECU/SoftECU/SRR_R/RearRight_SOD ==
  In1 : Inport
  Sensor_pos : Inport  Port=2
  CSP : Inport  Port=3
  Bus Creator : BusCreator  Inputs=4
  Bus Creator1 : BusCreator  Inputs=4
  Bus Creator2 : BusCreator  Inputs=4
  Bus Creator3 : BusCreator  Inputs=3
  Bus Selector : BusSelector  OutputSignals=SRR_R_DET_RANGE_01[m],SRR_R_DET_RANGE_RATE_01[m/s],SRR_R_DET_AZIMUTH_01[rad],SRR_R_DET_ELEVATION_01[rad]
  Bus Selector1 : BusSelector  OutputSignals=SRR_R_DET_RANGE_02[m],SRR_R_DET_RANGE_RATE_02[m/s],SRR_R_DET_AZIMUTH_02[rad],SRR_R_DET_ELEVATION_02[rad]
  Bus Selector2 : BusSelector  OutputSignals=SRR_R_DET_RANGE_03[m],SRR_R_DET_RANGE_RATE_03[m/s],SRR_R_DET_AZIMUTH_03[rad],SRR_R_DET_ELEVATION_03[rad]
  "SRR_RR_001 " : Subsystem
  SRR_RR_002 : Subsystem
  SRR_RR_003 : Subsystem
  RR_SOD : Outport
  wires:
  Bus Creator1/1 -> SRR_RR_002/1(target_pos)  "<Carsim_det_002>"
  Bus Selector1/3 -> Bus Creator1/3  "<SRR_R_DET_AZIMUTH_02[rad]>"
  Bus Creator/1 -> "SRR_RR_001 "/1(target_pos)  "<Carsim_det_001>"
  Bus Selector/2 -> Bus Creator/2  "<SRR_R_DET_RANGE_RATE_01[m/s]>"
  Bus Selector/1 -> Bus Creator/1  "<SRR_R_DET_RANGE_01[m]>"
  Bus Selector/4 -> Bus Creator/4  "<SRR_R_DET_ELEVATION_01[rad]>"
  Bus Selector/3 -> Bus Creator/3  "<SRR_R_DET_AZIMUTH_01[rad]>"
  Bus Selector1/1 -> Bus Creator1/1  "<SRR_R_DET_RANGE_02[m]>"
  Bus Selector2/2 -> Bus Creator2/2  "<SRR_R_DET_RANGE_RATE_03[m/s]>"
  Bus Selector1/2 -> Bus Creator1/2  "<SRR_R_DET_RANGE_RATE_02[m/s]>"
  Bus Selector2/1 -> Bus Creator2/1  "<SRR_R_DET_RANGE_03[m]>"
  In1/1 -> Bus Selector2/1, Bus Selector1/1, Bus Selector/1
  SRR_RR_003/1(SRR_RR_003) -> Bus Creator3/3  "SRR_RR_003"
  Bus Selector1/4 -> Bus Creator1/4  "<SRR_R_DET_ELEVATION_02[rad]>"
  Bus Selector2/3 -> Bus Creator2/3  "<SRR_R_DET_AZIMUTH_03[rad]>"
  Bus Selector2/4 -> Bus Creator2/4  "<SRR_R_DET_ELEVATION_03[rad]>"
  Bus Creator2/1 -> SRR_RR_003/1(target_pos)  "<Carsim_det_003>"
  Sensor_pos/1 -> SRR_RR_003/2(sensor_pos), SRR_RR_002/2(sensor_pos), "SRR_RR_001 "/2(sensor_pos)
  CSP/1 -> "SRR_RR_001 "/3(CSP), SRR_RR_003/3(CSP), SRR_RR_002/3(CSP)
  Bus Creator3/1 -> RR_SOD/1
  "SRR_RR_001 "/1(SRR_RR_001) -> Bus Creator3/1  "SRR_RR_001"
  SRR_RR_002/1(SRR_RR_002) -> Bus Creator3/2  "SRR_RR_002"

== system P702_NI_SoftECU/SoftECU/SRR_R/SensorPosition_FR ==
  note: Position in Carsim Coordinate
      | X: forward
      | Y: left
      | Lhan18
  Bus Creator : BusCreator  Inputs=3
  Gain1 : Gain  Gain=pi/180
  x_offset : Constant  Value=0.5
  y_offset : Constant  Value=-0.8
  yaw_head : Constant  Value=-60
  SensorPosition : Outport
  wires:
  Gain1/1 -> Bus Creator/3  "sensor_yaw"
  yaw_head/1 -> Gain1/1
  y_offset/1 -> Bus Creator/2  "sensor_y"
  x_offset/1 -> Bus Creator/1  "sensor_x"
  Bus Creator/1 -> SensorPosition/1  "Position"

== system P702_NI_SoftECU/SoftECU/SRR_R/SensorPosition_RR ==
  note: Position in Carsim Coordinate
      | X: forward
      | Y: left
      | Lhan18
  Bus Creator : BusCreator  Inputs=3
  Gain1 : Gain  Gain=pi/180
  x_offset : Constant  Value=-3.5
  y_offset : Constant  Value=-0.8
  yaw_head : Constant  Value=-120
  SensorPosition : Outport
  wires:
  Bus Creator/1 -> SensorPosition/1  "Position"
  x_offset/1 -> Bus Creator/1  "sensor_x"
  y_offset/1 -> Bus Creator/2  "sensor_y"
  yaw_head/1 -> Gain1/1
  Gain1/1 -> Bus Creator/3  "sensor_yaw"

== system P702_NI_SoftECU/SoftECU/TCM/Logic ==
  In1 : Inport
  Bus Creator3 : BusCreator  Inputs=1
  Bus Selector4 : BusSelector  OutputSignals=Gear_Lever_POS[]
  ReValueStates : Subsystem
      mask Display: disp('RevalueStates')
  Out1 : Outport
  wires:
  Bus Creator3/1 -> Out1/1  "LogicSignals"
  In1/1 -> Bus Selector4/1
  ReValueStates/1(Transmission_Ratio[-]) -> Bus Creator3/1  "GearLvrPos_D_ActlPart"
  Bus Selector4/1 -> ReValueStates/1(GearLvr[-])  "<Gear_Lever_POS[]>"

== system P702_NI_SoftECU/SoftECU/TCM/Mapping ==
  In1 : Inport
  Bus Creator1 : BusCreator  Inputs=1
  TransGearData : Subsystem
  Out1 : Outport
  wires:
  Bus Creator1/1 -> Out1/1  "MsgSignals"
  In1/1 -> TransGearData/1(In1)
  TransGearData/1(Out1) -> Bus Creator1/1  "TransGearData"

== system P702_NI_SoftECU/Input/Carsim/Bus Conversion/ABS_BUS ==
  In1 : Inport
  Bus Creator : BusCreator  Inputs=15
  Bus Selector : BusSelector  OutputSignals=Pos_Vehicle_GPS[long][deg],Pos_Vehicle_GPS[lat][deg],Omega_FL_wheel[rpm],Omega_FR_wheel[rpm],Omega_RL_wheel[rpm],Omega_RR_wheel[rpm],a_x_veh_COG[m/s2],a_y_veh_COG[m/s2],YawRate_Vehicle_COG[deg/s],V_total_Vehicle[km/h],a_z_Vehicle_COG[m/s2],RollRate_Vehicle_COG[deg/s],PitchRate_Vehicle_COG[deg/s],Angle_SteeringWheel[deg],Pos_BrakePedal[percentage]
  Gain : Gain  Gain=100
  Gain1 : Gain  Gain=9.8
  Gain2 : Gain  Gain=9.8
  Gain3 : Gain  Gain=9.8
  Out1 : Outport
  wires:
  In1/1 -> Bus Selector/1
  Gain3/1 -> Bus Creator/11  "a_z_Vehicle_COG[m/s2]"
  Gain2/1 -> Bus Creator/8  "a_y_veh_COG[m/s2]"
  Gain1/1 -> Bus Creator/7  "a_x_veh_COG[m/s2]"
  Gain/1 -> Bus Creator/15  "Pos_BrakePedal[percentage]"
  Bus Selector/5 -> Bus Creator/5  "<Omega_RL_wheel[rpm]>"
  Bus Selector/15 -> Gain/1  "<Pos_BrakePedal[percentage]>"
  Bus Selector/14 -> Bus Creator/14  "<Angle_SteeringWheel[deg]>"
  Bus Selector/8 -> Gain2/1  "<a_y_veh_COG[m/s2]>"
  Bus Selector/4 -> Bus Creator/4  "<Omega_FR_wheel[rpm]>"
  Bus Selector/6 -> Bus Creator/6  "<Omega_RR_wheel[rpm]>"
  Bus Selector/10 -> Bus Creator/10  "<V_total_Vehicle[km/h]>"
  Bus Selector/7 -> Gain1/1  "<a_x_veh_COG[m/s2]>"
  Bus Selector/1 -> Bus Creator/1  "<Pos_Vehicle_GPS[long][deg]>"
  Bus Selector/2 -> Bus Creator/2  "<Pos_Vehicle_GPS[lat][deg]>"
  Bus Selector/12 -> Bus Creator/12  "<RollRate_Vehicle_COG[deg/s]>"
  Bus Selector/3 -> Bus Creator/3  "<Omega_FL_wheel[rpm]>"
  Bus Selector/11 -> Gain3/1  "<a_z_Vehicle_COG[m/s2]>"
  Bus Selector/13 -> Bus Creator/13  "<PitchRate_Vehicle_COG[deg/s]>"
  Bus Selector/9 -> Bus Creator/9  "<YawRate_Vehicle_COG[deg/s]>"
  Bus Creator/1 -> Out1/1

== system P702_NI_SoftECU/Input/Carsim/Bus Conversion/ABS_BUS1 ==
  In1 : Inport
  Bus Creator : BusCreator  Inputs=15
  Bus Selector : BusSelector  OutputSignals=Pos_Vehicle_GPS[long][deg],Pos_Vehicle_GPS[lat][deg],Omega_FL_wheel[rpm],Omega_FR_wheel[rpm],Omega_RL_wheel[rpm],Omega_RR_wheel[rpm],a_x_veh_COG[m/s2],a_y_veh_COG[m/s2],YawRate_Vehicle_COG[deg/s],V_total_Vehicle[km/h],a_z_Vehicle_COG[m/s2],RollRate_Vehicle_COG[deg/s],PitchRate_Vehicle_COG[deg/s],Angle_SteeringWheel[deg],Pos_BrakePedal[percentage]
  Gain : Gain  Gain=100
  Gain{1..3,6..9} (7 alike) : Gain
  Gain{4..5,10,12..14} (6 alike) : Gain  Gain=180/pi
  Gain11 : Gain  Gain=3.6
  Out1 : Outport
  wires:
  In1/1 -> Bus Selector/1
  Gain3/1 -> Bus Creator/11  "a_z_Vehicle_COG[m/s2]"
  Gain2/1 -> Bus Creator/8  "a_y_veh_COG[m/s2]"
  Gain1/1 -> Bus Creator/7  "a_x_veh_COG[m/s2]"
  Gain/1 -> Bus Creator/15  "Pos_BrakePedal[percentage]"
  Bus Selector/5 -> Gain8/1  "<Omega_RL_wheel[rpm]>"
  Bus Selector/15 -> Gain/1  "<Pos_BrakePedal[percentage]>"
  Bus Selector/14 -> Gain14/1  "<Angle_SteeringWheel[deg]>"
  Bus Selector/8 -> Gain2/1  "<a_y_veh_COG[m/s2]>"
  Bus Selector/4 -> Gain7/1  "<Omega_FR_wheel[rpm]>"
  Bus Selector/6 -> Gain9/1  "<Omega_RR_wheel[rpm]>"
  Bus Selector/10 -> Gain11/1  "<V_total_Vehicle[km/h]>"
  Bus Selector/7 -> Gain1/1  "<a_x_veh_COG[m/s2]>"
  Bus Selector/1 -> Gain4/1  "<Pos_Vehicle_GPS[long][deg]>"
  Bus Selector/2 -> Gain5/1  "<Pos_Vehicle_GPS[lat][deg]>"
  Bus Selector/12 -> Gain12/1  "<RollRate_Vehicle_COG[deg/s]>"
  Bus Selector/3 -> Gain6/1  "<Omega_FL_wheel[rpm]>"
  Bus Selector/11 -> Gain3/1  "<a_z_Vehicle_COG[m/s2]>"
  Bus Selector/13 -> Gain13/1  "<PitchRate_Vehicle_COG[deg/s]>"
  Bus Selector/9 -> Gain10/1  "<YawRate_Vehicle_COG[deg/s]>"
  Bus Creator/1 -> Out1/1
  Gain4/1 -> Bus Creator/1  "Pos_Vehicle_GPS[long][deg]"
  Gain5/1 -> Bus Creator/2  "Pos_Vehicle_GPS[lat][deg]"
  Gain6/1 -> Bus Creator/3  "Omega_FL_wheel[rpm]"
  Gain7/1 -> Bus Creator/4  "Omega_FR_wheel[rpm]"
  Gain8/1 -> Bus Creator/5  "Omega_RL_wheel[rpm]"
  Gain9/1 -> Bus Creator/6  "Omega_RR_wheel[rpm]"
  Gain10/1 -> Bus Creator/9  "YawRate_Vehicle_COG[deg/s]"
  Gain11/1 -> Bus Creator/10  "V_total_Vehicle[km/h]"
  Gain12/1 -> Bus Creator/12  "RollRate_Vehicle_COG[deg/s]"
  Gain13/1 -> Bus Creator/13  "PitchRate_Vehicle_COG[deg/s]"
  Gain14/1 -> Bus Creator/14  "Angle_SteeringWheel[deg]"

== system P702_NI_SoftECU/Input/Carsim/Bus Conversion/BCM_BUS ==
  In1 : Inport
  Bus Creator : BusCreator  Inputs=1
  Bus Selector : BusSelector  OutputSignals=s_Vehicle[m]
  Out1 : Outport
  wires:
  Bus Creator/1 -> Out1/1
  Bus Selector/1 -> Bus Creator/1  "<s_Vehicle[m]>"
  In1/1 -> Bus Selector/1

== system P702_NI_SoftECU/Input/Carsim/Bus Conversion/BCM_BUS1 ==
  In1 : Inport
  Bus Creator : BusCreator  Inputs=1
  Bus Selector : BusSelector  OutputSignals=s_Vehicle[m]
  Out1 : Outport
  wires:
  Bus Creator/1 -> Out1/1
  Bus Selector/1 -> Bus Creator/1  "<s_Vehicle[m]>"
  In1/1 -> Bus Selector/1

== system P702_NI_SoftECU/Input/Carsim/Bus Conversion/ECM_BUS ==
  In1 : Inport
  Bus Creator : BusCreator  Inputs=2
  Bus Selector : BusSelector  OutputSignals=Engine_RPM[rpm],V_x_veh_COG[km/h]
  Out1 : Outport
  wires:
  Bus Selector/2 -> Bus Creator/2  "<V_x_veh_COG[km/h]>"
  Bus Creator/1 -> Out1/1
  Bus Selector/1 -> Bus Creator/1  "<Engine_RPM[rpm]>"
  In1/1 -> Bus Selector/1

== system P702_NI_SoftECU/Input/Carsim/Bus Conversion/ECM_BUS1 ==
  note: g
  In1 : Inport
  Bus Creator : BusCreator  Inputs=2
  Bus Selector : BusSelector  OutputSignals=Engine_RPM[rpm],V_x_veh_COG[km/h]
  Gain : Gain  Gain=30/pi
  Gain1 : Gain  Gain=3.6
  Out1 : Outport
  wires:
  Bus Selector/2 -> Gain1/1  "<V_x_veh_COG[km/h]>"
  Bus Creator/1 -> Out1/1
  Bus Selector/1 -> Gain/1  "<Engine_RPM[rpm]>"
  In1/1 -> Bus Selector/1
  Gain/1 -> Bus Creator/1  "Engine_RPM[rpm]"
  Gain1/1 -> Bus Creator/2  "V_x_veh_COG[km/h]"

== system P702_NI_SoftECU/Input/Carsim/Bus Conversion/GPSM_BUS ==
  In1 : Inport
  Bus Creator : BusCreator  Inputs=5
  Bus Selector : BusSelector  OutputSignals=Pos_Z_veh[m],Pos_veh_long[deg],Pos_veh_lat[deg],Angle_Yaw_veh[deg],V_total_veh
  Out1 : Outport
  wires:
  Bus Creator/1 -> Out1/1
  In1/1 -> Bus Selector/1
  Bus Selector/5 -> Bus Creator/5  "<V_total_veh>"
  Bus Selector/4 -> Bus Creator/4  "<Angle_Yaw_veh[deg]>"
  Bus Selector/3 -> Bus Creator/3  "<Pos_veh_lat[deg]>"
  Bus Selector/2 -> Bus Creator/2  "<Pos_veh_long[deg]>"
  Bus Selector/1 -> Bus Creator/1  "<Pos_Z_veh[m]>"

== system P702_NI_SoftECU/Input/Carsim/Bus Conversion/GPSM_BUS1 ==
  In1 : Inport
  Bus Creator : BusCreator  Inputs=5
  Bus Selector : BusSelector  OutputSignals=Pos_Z_veh[m],Pos_veh_long[deg],Pos_veh_lat[deg],Angle_Yaw_veh[deg],V_total_veh
  Out1 : Outport
  wires:
  Bus Creator/1 -> Out1/1
  In1/1 -> Bus Selector/1
  Bus Selector/5 -> Bus Creator/5  "<V_total_veh>"
  Bus Selector/4 -> Bus Creator/4  "<Angle_Yaw_veh[deg]>"
  Bus Selector/3 -> Bus Creator/3  "<Pos_veh_lat[deg]>"
  Bus Selector/2 -> Bus Creator/2  "<Pos_veh_long[deg]>"
  Bus Selector/1 -> Bus Creator/1  "<Pos_Z_veh[m]>"

== system P702_NI_SoftECU/Input/Carsim/Bus Conversion/MRR_BUS ==
  In1 : Inport
  Bus Creator : BusCreator  Inputs=12
  Bus Selector : BusSelector  OutputSignals=CAN_DET_RANGE_01[m],CAN_DET_RANGE_RATE_01[m/s],CAN_DET_AZIMUTH_01[rad],CAN_DET_ELEVATION_01[rad],CAN_DET_RANGE_02[m],CAN_DET_RANGE_RATE_02[m/s],CAN_DET_AZIMUTH_02[rad],CAN_DET_ELEVATION_02[rad],CAN_DET_RANGE_03[m],CAN_DET_RANGE_RATE_03[m/s],CAN_DET_AZIMUTH_03[rad],CAN_DET_ELEVATION_03[rad]
  Gain : Gain  Gain=1/3.6
  Gain10 : Gain  Gain=pi/180
  Gain11 : Gain  Gain=-pi/180
  Gain12 : Gain  Gain=1/3.6
  Gain13 : Gain  Gain=-pi/180
  Gain14 : Gain  Gain=1/3.6
  Gain3 : Gain  Gain=-pi/180
  Gain6 : Gain  Gain=pi/180
  Gain9 : Gain  Gain=pi/180
  Out1 : Outport
  wires:
  Bus Selector/1 -> Bus Creator/1  "<CAN_DET_RANGE_01[m]>"
  Bus Selector/11 -> Gain11/1  "<CAN_DET_AZIMUTH_03[rad]>"
  Bus Selector/3 -> Gain3/1  "<CAN_DET_AZIMUTH_01[rad]>"
  Bus Selector/2 -> Gain/1  "<CAN_DET_RANGE_RATE_01[m/s]>"
  Bus Selector/7 -> Gain13/1  "<CAN_DET_AZIMUTH_02[rad]>"
  Bus Selector/6 -> Gain14/1  "<CAN_DET_RANGE_RATE_02[m/s]>"
  Bus Selector/9 -> Bus Creator/9  "<CAN_DET_RANGE_03[m]>"
  Bus Selector/5 -> Bus Creator/5  "<CAN_DET_RANGE_02[m]>"
  Bus Creator/1 -> Out1/1
  In1/1 -> Bus Selector/1
  Bus Selector/4 -> Gain10/1  "<CAN_DET_ELEVATION_01[rad]>"
  Bus Selector/12 -> Gain6/1  "<CAN_DET_ELEVATION_03[rad]>"
  Bus Selector/8 -> Gain9/1  "<CAN_DET_ELEVATION_02[rad]>"
  Gain/1 -> Bus Creator/2  "CAN_DET_RANGE_RATE_01[m/s]"
  Gain3/1 -> Bus Creator/3  "CAN_DET_AZIMUTH_01[rad]"
  Gain10/1 -> Bus Creator/4  "CAN_DET_ELEVATION_01[rad]"
  Gain14/1 -> Bus Creator/6  "CAN_DET_RANGE_RATE_02[m/s]"
  Gain13/1 -> Bus Creator/7  "CAN_DET_AZIMUTH_02[rad]"
  Gain9/1 -> Bus Creator/8  "CAN_DET_ELEVATION_02[rad]"
  Gain12/1 -> Bus Creator/10  "CAN_DET_RANGE_RATE_03[m/s]"
  Gain11/1 -> Bus Creator/11  "CAN_DET_AZIMUTH_03[rad]"
  Gain6/1 -> Bus Creator/12  "CAN_DET_ELEVATION_03[rad]"
  Bus Selector/10 -> Gain12/1  "<CAN_DET_RANGE_RATE_03[m/s]>"
